simulink model "Gravity_Compensate"  (R2018b)
settings: Solver=FixedStepAuto  StartTime=0.0  StopTime=inf  FixedStep=0.001  RelTol=1e-3  EnableMultiTasking=on
values from neighbouring files (symbols this model uses):
  Dis_Coff = [0.42361 0.19319 -26.689 1.2064 -2.9972 4045.7 -3.3883 3.6846 291430]    [Robot_Parameters_Ident_With_Disturbance.mat]
  F1G = 0.2    [Main_Code.m]    (also in Main_Code_Gravity_Compensation.m)
  F2G = 0.2    [Main_Code.m]    (also in Main_Code_Gravity_Compensation.m)
  F3G = 0.005    [Main_Code.m]    (also in Main_Code_Gravity_Compensation.m)
  phi_Dynamic = [phi0;phi1;phi2;phi3;phi4;phi5;phi6;phi7]    [Parameters_Builder.m]    (also in Robot_Parameters.mat = [0.73163251 -0.0393 0 2.40643096032e-18 0.000785329049449 0.; Robot_Parameters_Ident.mat = [0.78122 -0.0393 0 2.40643096032e-18 0.000785329049449 0.000; Robot_Parameters_Ident_With_Disturbance.mat = [0.78122 -0.0393 0 2.40643096032e-18 0.000785329049449 0.000)
  phi_Kinematic = [l__0;l__1;l__3;l__5;l__2;l__7;theta;alpha;d__0;l__x35;l__z35;psi0]    [Parameters_Builder.m]    (also in Robot_Parameters.mat = [0.006 0.182 0.05 0.115 0.07 0.0342 0.733038285838 0.8726646; Robot_Parameters_Ident.mat = [0.006 0.182 0.05 0.115 0.07 0.0342 0.733038285838 0.8726646; Robot_Parameters_Ident_With_Disturbance.mat = [0.006 0.182 0.05 0.115 0.07 0.0342 0.733038285838 0.8726646)
libraries: neural x94, xpcrtudplib x3, xpcutilitieslib x2, slrtlib x1
(part 1 of 3)
settings Model: SimulationMode=external  Creator=ARAS  LastModifiedBy=ARAS
settings SolverCC: ConcurrentTasks=on  AutoInsertRateTranBlk=on
settings DataIOCC: SaveFormat=StructureWithTime
settings OptimizationCC: BlockReduction=off  OptimizeBlockIOStorage=off  BufferReuse=off  GlobalBufferReuse=off  ExpressionFolding=off  LocalBlockOutputs=off  OptimizeDataStoreBuffers=off  BusAssignmentInplaceUpdate=off
settings HardwareCC: ProdBitPerPointer=32  ProdBitPerSizeT=32  ProdBitPerPtrDiffT=32  ProdLargestAtomicFloat=None  ProdWordSize=32  ProdLongLongMode=on  ProdHWDeviceType=Generic->32-bit x86 compatible
settings RTWCC: SystemTargetFile=slrt.tlc  TemplateMakefile=slrt_default_tmf  Description=Simulink Real-Time  CodeExecutionProfiling=on  RTWCompilerOptimization=on
settings SimulinkRealTimeCC: SupportVariableSizeSignals=on  PreserveStateflowLocalDataDimensions=off  RL32LogTETModifier=off  xPCConcurrentTasks=on

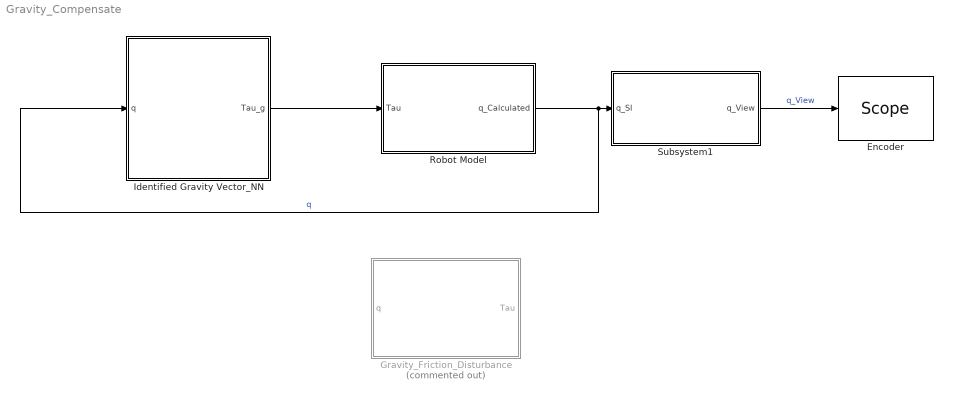
== system Gravity_Compensate ==
  Encoder : slrtlib/Displays and Logging/Scope   scopeno=2  scopetype=Target  autostart=on  viewmode=Numerical  formatstr='%15.6f'  grid=on  ylimits=[0,0]  nosamples=3  noprepostsamples=0  interleave=1  triggermode=FreeRun  triggersignal=1  trigsignalfromport=off  triggerlevel=0.0  triggerslope=Either  triggerscope=1  triggersample=0  filename=data.dat  mode=Lazy  writesize=512  autorestart=off  dynamicfilemode=off  maxwritefilesize=512*1024^2
  Gravity_Friction_Disturbance : Subsystem  Commented=on
  Identified Gravity Vector_NN : Subsystem
  Robot Model : Subsystem
  Subsystem1 : Subsystem
  wires:
  Subsystem1/1(q_View) -> Encoder/1  "q_View"
  Robot Model/1(q_Calculated) -> Identified Gravity Vector_NN/1(q), Subsystem1/1(q_SI)  "q"
  Identified Gravity Vector_NN/1(Tau_g) -> Robot Model/1(Tau)

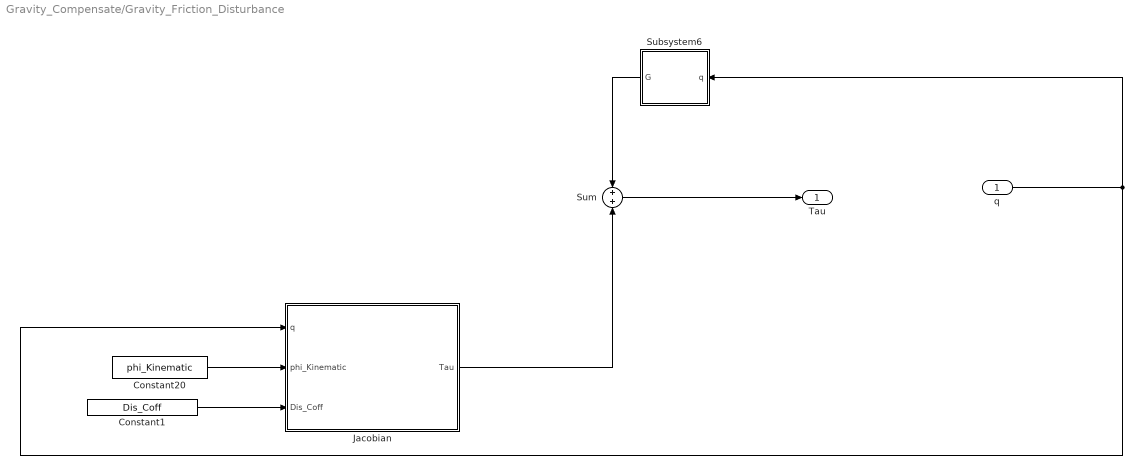
== system Gravity_Compensate/Gravity_Friction_Disturbance ==
  q : Inport
  Constant1 : Constant  Value=Dis_Coff
  Constant20 : Constant  Value=phi_Kinematic
  Jacobian : MATLAB Function  TreatAsAtomicUnit=on
  Subsystem6 : Subsystem
  Sum : Sum  Inputs=+|+
  Tau : Outport
  wires:
  q/1 -> Jacobian/1(q), Subsystem6/1(q)
  Constant1/1 -> Jacobian/3(Dis_Coff)
  Jacobian/1(Tau) -> Sum/2
  Constant20/1 -> Jacobian/2(phi_Kinematic)
  Subsystem6/1(G) -> Sum/1
  Sum/1 -> Tau/1

== system Gravity_Compensate/Identified Gravity Vector_NN ==
  q : Inport
  High_Epoch_Model : Subsystem
      mask help: Function Fitting Neural Network
      mask Display: e = 0.06;c1 = [120 150 230]/255;c2 = ([120 150 230]+0)/383;c3 = ([120 150 230]+128)/383;patch([0 1 1 0],[0 0 1 1],c1);patch([0 1 1 1-e 1-e 0+e],[0 0 1 1-e 0+e 0+e],c2);patch([0 0 1 1-e 0+e 0+e],[0 1 1 1-e 1-e 0+e],c3);plot([0 1 1 0 0],[0 0 1 1 0]);fprintf('NNET');port_label('input',1,' Input');port_label('output',1,'Output ');
  Simple_Model : Subsystem  Commented=on
      mask help: Function Fitting Neural Network
      mask Display: e = 0.06;c1 = [120 150 230]/255;c2 = ([120 150 230]+0)/383;c3 = ([120 150 230]+128)/383;patch([0 1 1 0],[0 0 1 1],c1);patch([0 1 1 1-e 1-e 0+e],[0 0 1 1-e 0+e 0+e],c2);patch([0 0 1 1-e 0+e 0+e],[0 1 1 1-e 1-e 0+e],c3);plot([0 1 1 0 0],[0 0 1 1 0]);fprintf('NNET');port_label('input',1,' Input');port_label('output',1,'Output ');
  Tau_g : Outport
  wires:
  High_Epoch_Model/1(Output) -> Tau_g/1
  q/1 -> High_Epoch_Model/1(Input)

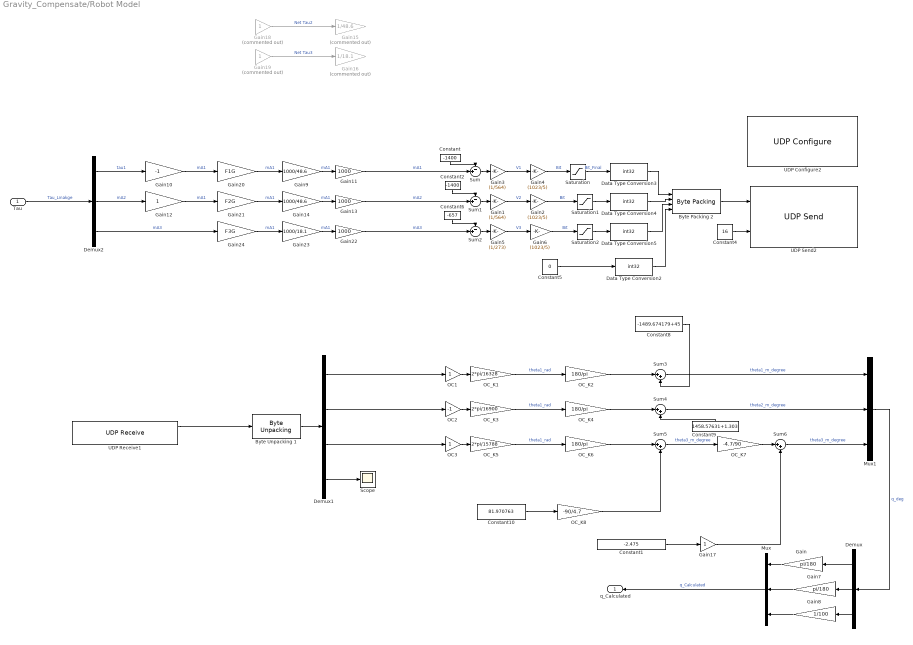
== system Gravity_Compensate/Robot Model ==
  Tau : Inport
  Byte Packing 2 : xpcutilitieslib/Byte Packing   MaskPackedDataType=uint8  MaskUnpackedDataTypes={'int32','int32','int32','int32'}  MaskAlignment=1
  Byte Unpacking 1 : xpcutilitieslib/Byte Unpacking   MaskUnpackedDataTypes={'int32'}  MaskUnpackedDataSizes={[4]}  MaskAlignment=1
      settings: SourceProductName=Simulink Real-Time  SourceProductBaseCode=XP
  Constant : Constant  Value=-1400
  Constant1 : Constant  Value=-2.475
  Constant10 : Constant  Value=81.970763
  Constant2 : Constant  Value=-1400
  Constant4 : Constant  Value=16
  Constant5 : Constant  Value=0
  Constant6 : Constant  Value=-657
  Constant8 : Constant  Value=-1489.674179+45
  Constant9 : Constant  Value=1458.57631+1.303
  Data Type Conversion{2..5} (4 alike) : DataTypeConversion  OutDataTypeStr=int32
  Demux : Demux  Outputs=3
  Demux1 : Demux
  Demux2 : Demux  Outputs=3
  Gain : Gain  Gain=pi/180
  Gain1 : Gain  Gain=(1/564)
  Gain10 : Gain  Gain=-1
  Gain11 : Gain  Gain=1000
  Gain12 : Gain
  Gain13 : Gain  Gain=1000
  Gain14 : Gain  Gain=1000/48.6
  Gain15 : Gain  Commented=on  Gain=1/48.6
  Gain16 : Gain  Commented=on  Gain=1/18.1
  Gain17 : Gain
  Gain18 : Gain  Commented=on
  Gain19 : Gain  Commented=on
  Gain2 : Gain  Gain=(1023/5)
  Gain20 : Gain  Gain=F1G
  Gain21 : Gain  Gain=F2G
  Gain22 : Gain  Gain=1000
  Gain23 : Gain  Gain=1000/18.1
  Gain24 : Gain  Gain=F3G
  Gain3 : Gain  Gain=(1/564)
  Gain4 : Gain  Gain=(1023/5)
  Gain5 : Gain  Gain=(1/273)
  Gain6 : Gain  Gain=(1023/5)
  Gain7 : Gain  Gain=pi/180
  Gain8 : Gain  Gain=1/100
  Gain9 : Gain  Gain=1000/48.6
  Mux : Mux  Inputs=3
  Mux1 : Mux  Inputs=3
  OC1 : Gain  ParamDataTypeStr=double  OutDataTypeStr=double
  OC2 : Gain  Gain=-1  ParamDataTypeStr=double  OutDataTypeStr=double
  OC3 : Gain  ParamDataTypeStr=double  OutDataTypeStr=double
  OC_K1 : Gain  Gain=2*pi/16328  ParamDataTypeStr=double  OutDataTypeStr=double
  OC_K2 : Gain  Gain=180/pi  ParamDataTypeStr=double  OutDataTypeStr=double
  OC_K3 : Gain  Gain=2*pi/16900  ParamDataTypeStr=double  OutDataTypeStr=double
  OC_K4 : Gain  Gain=180/pi  ParamDataTypeStr=double  OutDataTypeStr=double
  OC_K5 : Gain  Gain=2*pi/15788  ParamDataTypeStr=double  OutDataTypeStr=double
  OC_K6 : Gain  Gain=180/pi  ParamDataTypeStr=double  OutDataTypeStr=double
  OC_K7 : Gain  Gain=-4.7/90  ParamDataTypeStr=double  OutDataTypeStr=double
  OC_K8 : Gain  Gain=-90/4.7  ParamDataTypeStr=double  OutDataTypeStr=double
  Saturation : Saturate  UpperLimit=1023  LowerLimit=0
  Saturation1 : Saturate  UpperLimit=1023  LowerLimit=0
  Saturation2 : Saturate  UpperLimit=1023  LowerLimit=0
  Scope : Scope
  Sum : Sum  Inputs=-+|
  Sum1 : Sum  Inputs=-+|
  Sum2 : Sum  Inputs=-+|
  Sum{3..6} (4 alike) : Sum  Inputs=|++
  UDP Configure2 : xpcrtudplib/UDP Configure  Priority=-1  IpAddress=192.168.1.4  SubnetMask=255.255.255.0  Gateway=0.0.0.0  PciBus=[3]  PciSlot=[1]  PciFunction=0  ID=1  tune=0  disable=off  enableMulticast=off  MulticastIpAddress={}  MulticastMask={}
      settings: SourceProductName=Simulink Real-Time  SourceProductBaseCode=XP
  UDP Receive1 : xpcrtudplib/UDP Receive  ipAddressVal=192.168.1.4  localPort=5500  rcvWidth=16  rcvFmAny=on  fmAddress=0.0.0.0  rcvMulticast=off  multicastAddress={}  maxUDPQueue=8  sampleTime=0.001
      settings: SourceProductName=Simulink Real-Time
  UDP Send2 : xpcrtudplib/UDP Send  ipAddressVal=192.168.1.4  localPort=5500  toAddress=192.168.1.3  toPort=5500  sampleTime=0.001
      settings: SourceProductName=Simulink Real-Time  SourceProductBaseCode=XP
  q_Calculated : Outport
  wires:
  Demux1/2 -> OC2/1
  Sum/1 -> Gain3/1
  Data Type Conversion2/1 -> Byte Packing 2/4
  OC_K1/1 -> OC_K2/1  "theta1_rad"
  Byte Packing 2/1 -> UDP Send2/1
  Gain4/1 -> Saturation/1  "Bit"
  OC1/1 -> OC_K1/1
  Constant4/1 -> UDP Send2/2
  UDP Receive1/1 -> Byte Unpacking 1/1
  OC_K2/1 -> Sum3/1
  Data Type Conversion3/1 -> Byte Packing 2/1
  Data Type Conversion4/1 -> Byte Packing 2/2
  Data Type Conversion5/1 -> Byte Packing 2/3
  Demux1/3 -> OC3/1
  Constant5/1 -> Data Type Conversion2/1
  OC_K4/1 -> Sum4/1
  Constant/1 -> Sum/1
  Saturation/1 -> Data Type Conversion3/1  "Bit_Final"
  Constant10/1 -> OC_K8/1
  Gain3/1 -> Gain4/1  "V1"
  OC_K6/1 -> Sum5/1
  Saturation2/1 -> Data Type Conversion5/1
  Constant6/1 -> Sum2/1
  Gain6/1 -> Saturation2/1  "Bit"
  Gain5/1 -> Gain6/1  "V3"
  Sum2/1 -> Gain5/1
  Byte Unpacking 1/1 -> Demux1/1
  Sum1/1 -> Gain1/1
  Sum4/1 -> Mux1/2  "theta2_m_degree"
  Demux1/1 -> OC1/1
  Mux1/1 -> Demux/1  "q_deg"
  OC_K3/1 -> OC_K4/1  "theta1_rad"
  OC_K5/1 -> OC_K6/1  "theta1_rad"
  OC3/1 -> OC_K5/1
  Gain2/1 -> Saturation1/1  "Bit"
  Demux/1 -> Gain/1
  Tau/1 -> Demux2/1  "Tau_Linakge"
  Gain/1 -> Mux/1
  OC2/1 -> OC_K3/1
  Sum3/1 -> Mux1/1  "theta1_m_degree"
  Demux1/4 -> Scope/1
  Demux/2 -> Gain7/1
  Gain1/1 -> Gain2/1  "V2"
  Gain7/1 -> Mux/2
  Constant8/1 -> Sum3/2
  Constant9/1 -> Sum4/2
  Constant2/1 -> Sum1/1
  Saturation1/1 -> Data Type Conversion4/1
  Mux/1 -> q_Calculated/1  "q_Calculated"
  Gain18/1 -> Gain15/1  "Net Tau2"
  Gain19/1 -> Gain16/1  "Net Tau3"
  Demux2/1 -> Gain10/1  "tau1"
  Gain9/1 -> Gain11/1  "mA1"
  Gain10/1 -> Gain20/1  "mA1"
  Gain11/1 -> Sum/2  "mA1"
  Gain14/1 -> Gain13/1  "mA1"
  Gain12/1 -> Gain21/1  "mA1"
  Gain13/1 -> Sum1/2  "mA2"
  Demux2/2 -> Gain12/1  "mA2"
  Demux/3 -> Gain8/1
  Gain8/1 -> Mux/3
  Gain23/1 -> Gain22/1  "mA1"
  Gain22/1 -> Sum2/2  "mA3"
  Demux2/3 -> Gain24/1  "mA3"
  OC_K8/1 -> Sum5/2
  Sum5/1 -> OC_K7/1  "theta3_m_degree"
  OC_K7/1 -> Sum6/1
  Sum6/1 -> Mux1/3  "theta3_m_degree"
  Constant1/1 -> Gain17/1
  Gain17/1 -> Sum6/2
  Gain20/1 -> Gain9/1  "mA1"
  Gain21/1 -> Gain14/1  "mA1"
  Gain24/1 -> Gain23/1  "mA1"

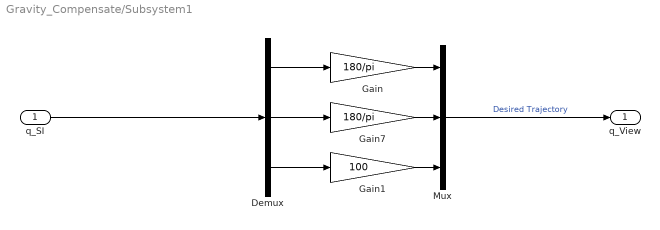
== system Gravity_Compensate/Subsystem1 ==
  q_SI : Inport
  Demux : Demux  Outputs=3
  Gain : Gain  Gain=180/pi
  Gain1 : Gain  Gain=100
  Gain7 : Gain  Gain=180/pi
  Mux : Mux  Inputs=3
  q_View : Outport
  wires:
  Gain7/1 -> Mux/2
  Demux/3 -> Gain1/1
  Demux/2 -> Gain7/1
  q_SI/1 -> Demux/1
  Gain/1 -> Mux/1
  Demux/1 -> Gain/1
  Mux/1 -> q_View/1  "Desired Trajectory"
  Gain1/1 -> Mux/3

== system Gravity_Compensate/Gravity_Friction_Disturbance/Subsystem6 ==
  q : Inport
  Constant : Constant  Value=phi_Kinematic
  Constant4 : Constant  Value=phi_Dynamic
  MATLAB Function1 : MATLAB Function  TreatAsAtomicUnit=on
  G : Outport
  wires:
  q/1 -> MATLAB Function1/1(q)
  MATLAB Function1/1(G) -> G/1
  Constant4/1 -> MATLAB Function1/3(phi_Dynamic)
  Constant/1 -> MATLAB Function1/2(phi_Kinematic)

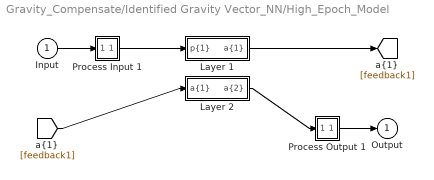
== system Gravity_Compensate/Identified Gravity Vector_NN/High_Epoch_Model ==
  Input : Inport  PortDimensions=3
      mask Display: e = 0.06;c1 = [120 230 180]/255;c2 = ([120 230 180]+0)/(256+128);c3 = ([120 230 180]+128)/(256+128);patch([0 1 1 0],[0 0 1 1],c1);patch([0 1 1 1-e 1-e 0+e],[0 0 1 1-e 0+e 0+e],c2);patch([0 0 1 1-e 0+e 0+e],[0 1 1 1-e 1-e 0+e],c3);plot([0 1 1 0 0],[0 0 1 1 0]);
  Layer 1 : Subsystem
      mask Display: e = 0.06;c1 = [120 150 230]/255;c2 = ([120 150 230]+0)/383;c3 = ([120 150 230]+128)/383;patch([0 1 1 0],[0 0 1 1],c1);patch([0 1 1 1-e 1-e 0+e],[0 0 1 1-e 0+e 0+e],c2);patch([0 0 1 1-e 0+e 0+e],[0 1 1 1-e 1-e 0+e],c3);plot([0 1 1 0 0],[0 0 1 1 0]);
  Layer 2 : Subsystem
      mask Display: e = 0.06;c1 = [120 150 230]/255;c2 = ([120 150 230]+0)/383;c3 = ([120 150 230]+128)/383;patch([0 1 1 0],[0 0 1 1],c1);patch([0 1 1 1-e 1-e 0+e],[0 0 1 1-e 0+e 0+e],c2);patch([0 0 1 1-e 0+e 0+e],[0 1 1 1-e 1-e 0+e],c3);plot([0 1 1 0 0],[0 0 1 1 0]);
  Process Input 1 : Subsystem
      mask Display: e = 0.06;c1 = [120 150 230]/255;c2 = ([120 150 230]+0)/383;c3 = ([120 150 230]+128)/383;patch([0 1 1 0],[0 0 1 1],c1);patch([0 1 1 1-e 1-e 0+e],[0 0 1 1-e 0+e 0+e],c2);patch([0 0 1 1-e 0+e 0+e],[0 1 1 1-e 1-e 0+e],c3);plot([0 1 1 0 0],[0 0 1 1 0]);
  Process Output 1 : Subsystem
      mask Display: e = 0.06;c1 = [120 150 230]/255;c2 = ([120 150 230]+0)/383;c3 = ([120 150 230]+128)/383;patch([0 1 1 0],[0 0 1 1],c1);patch([0 1 1 1-e 1-e 0+e],[0 0 1 1-e 0+e 0+e],c2);patch([0 0 1 1-e 0+e 0+e],[0 1 1 1-e 1-e 0+e],c3);plot([0 1 1 0 0],[0 0 1 1 0]);
  Output : Outport  InitialOutput=[0;0;0]
      mask Display: e = 0.06;c1 = [120 230 180]/255;c2 = ([120 230 180]+0)/(256+128);c3 = ([120 230 180]+128)/(256+128);patch([0 1 1 0],[0 0 1 1],c1);patch([0 1 1 1-e 1-e 0+e],[0 0 1 1-e 0+e 0+e],c2);patch([0 0 1 1-e 0+e 0+e],[0 1 1 1-e 1-e 0+e],c3);plot([0 1 1 0 0],[0 0 1 1 0]);
  wires:
  Input/1 -> Process Input 1/1(x)
  Process Output 1/1(y) -> Output/1
  Process Input 1/1(p) -> Layer 1/1("p{1}")
  Layer 1/1("a{1}") -> [feedback1]
  [feedback1] -> Layer 2/1("a{1} ")
  Layer 2/1("a{2}") -> Process Output 1/1(a)

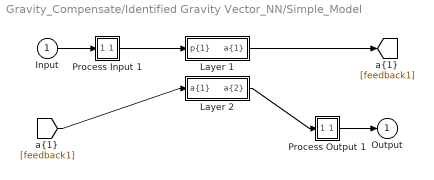
== system Gravity_Compensate/Identified Gravity Vector_NN/Simple_Model ==
  Input : Inport  PortDimensions=3
      mask Display: e = 0.06;c1 = [120 230 180]/255;c2 = ([120 230 180]+0)/(256+128);c3 = ([120 230 180]+128)/(256+128);patch([0 1 1 0],[0 0 1 1],c1);patch([0 1 1 1-e 1-e 0+e],[0 0 1 1-e 0+e 0+e],c2);patch([0 0 1 1-e 0+e 0+e],[0 1 1 1-e 1-e 0+e],c3);plot([0 1 1 0 0],[0 0 1 1 0]);
  Layer 1 : Subsystem
      mask Display: e = 0.06;c1 = [120 150 230]/255;c2 = ([120 150 230]+0)/383;c3 = ([120 150 230]+128)/383;patch([0 1 1 0],[0 0 1 1],c1);patch([0 1 1 1-e 1-e 0+e],[0 0 1 1-e 0+e 0+e],c2);patch([0 0 1 1-e 0+e 0+e],[0 1 1 1-e 1-e 0+e],c3);plot([0 1 1 0 0],[0 0 1 1 0]);
  Layer 2 : Subsystem
      mask Display: e = 0.06;c1 = [120 150 230]/255;c2 = ([120 150 230]+0)/383;c3 = ([120 150 230]+128)/383;patch([0 1 1 0],[0 0 1 1],c1);patch([0 1 1 1-e 1-e 0+e],[0 0 1 1-e 0+e 0+e],c2);patch([0 0 1 1-e 0+e 0+e],[0 1 1 1-e 1-e 0+e],c3);plot([0 1 1 0 0],[0 0 1 1 0]);
  Process Input 1 : Subsystem
      mask Display: e = 0.06;c1 = [120 150 230]/255;c2 = ([120 150 230]+0)/383;c3 = ([120 150 230]+128)/383;patch([0 1 1 0],[0 0 1 1],c1);patch([0 1 1 1-e 1-e 0+e],[0 0 1 1-e 0+e 0+e],c2);patch([0 0 1 1-e 0+e 0+e],[0 1 1 1-e 1-e 0+e],c3);plot([0 1 1 0 0],[0 0 1 1 0]);
  Process Output 1 : Subsystem
      mask Display: e = 0.06;c1 = [120 150 230]/255;c2 = ([120 150 230]+0)/383;c3 = ([120 150 230]+128)/383;patch([0 1 1 0],[0 0 1 1],c1);patch([0 1 1 1-e 1-e 0+e],[0 0 1 1-e 0+e 0+e],c2);patch([0 0 1 1-e 0+e 0+e],[0 1 1 1-e 1-e 0+e],c3);plot([0 1 1 0 0],[0 0 1 1 0]);
  Output : Outport  InitialOutput=[0;0;0]
      mask Display: e = 0.06;c1 = [120 230 180]/255;c2 = ([120 230 180]+0)/(256+128);c3 = ([120 230 180]+128)/(256+128);patch([0 1 1 0],[0 0 1 1],c1);patch([0 1 1 1-e 1-e 0+e],[0 0 1 1-e 0+e 0+e],c2);patch([0 0 1 1-e 0+e 0+e],[0 1 1 1-e 1-e 0+e],c3);plot([0 1 1 0 0],[0 0 1 1 0]);
  wires:
  Input/1 -> Process Input 1/1(x)
  Process Output 1/1(y) -> Output/1
  Process Input 1/1(p) -> Layer 1/1("p{1}")
  Layer 1/1("a{1}") -> [feedback1]
  [feedback1] -> Layer 2/1("a{1} ")
  Layer 2/1("a{2}") -> Process Output 1/1(a)

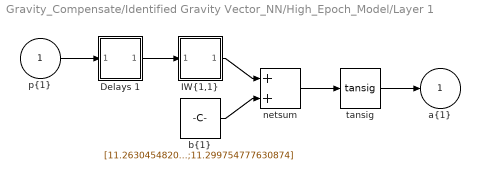
== system Gravity_Compensate/Identified Gravity Vector_NN/High_Epoch_Model/Layer 1 ==
  "p{1}" : Inport  PortDimensions=3
      mask Display: e = 0.06;c1 = [120 230 180]/255;c2 = ([120 230 180]+0)/(256+128);c3 = ([120 230 180]+128)/(256+128);patch([0 1 1 0],[0 0 1 1],c1);patch([0 1 1 1-e 1-e 0+e],[0 0 1 1-e 0+e 0+e],c2);patch([0 0 1 1-e 0+e 0+e],[0 1 1 1-e 1-e 0+e],c3);plot([0 1 1 0 0],[0 0 1 1 0]);
  Delays 1 : Subsystem
      mask Display: e = 0.06;c1 = [120 150 230]/255;c2 = ([120 150 230]+0)/383;c3 = ([120 150 230]+128)/383;patch([0 1 1 0],[0 0 1 1],c1);patch([0 1 1 1-e 1-e 0+e],[0 0 1 1-e 0+e 0+e],c2);patch([0 0 1 1-e 0+e 0+e],[0 1 1 1-e 1-e 0+e],c3);plot([0 1 1 0 0],[0 0 1 1 0]);disp('0');
  "IW{1,1}" : Subsystem
      mask Display: e = 0.06;c1 = [120 150 230]/255;c2 = ([120 150 230]+0)/383;c3 = ([120 150 230]+128)/383;patch([0 1 1 0],[0 0 1 1],c1);patch([0 1 1 1-e 1-e 0+e],[0 0 1 1-e 0+e 0+e],c2);patch([0 0 1 1-e 0+e 0+e],[0 1 1 1-e 1-e 0+e],c3);plot([0 1 1 0 0],[0 0 1 1 0]);disp('W');
  "b{1}" : Constant  Value=[11.263045482018567;6.0317742252947308;11.983996589226004;-7.6658588988543306;-5.8517886110739861;7.4451232310533406;10.917180640306658;-6.5870241683654687;8.0108681985756007;3.5513473095849979;9.6220293843375355;9.8565293533281011;3.5197166429287239;3.6957386521181124;5.6440514639510049;-3.0703225818481172;2.1993404217161325;-0.066943861917433428;-2.0448856298648423;1.6124187771848024;-0.018250185149015798;3.6417819857003435;-4.3109465870083543;-3.0890929292081832;3.9452928405896164;-5.6095743252511374;6.5578953711868264;4.3644627799494344;4.4419180604905453;7.0119603370043402;5.8581916985606002;6.7924155913571704;9.2191096669671992;-7.7729809830225198;-2.8799575409002096;-7.1021222037015077;8.151184925844742;-4.0986683409814439;9.8356397770443831;11.299754777630874]
      mask Display: e = 0.06;c1 = [120 150 230]/255;c2 = ([120 150 230]+0)/383;c3 = ([120 150 230]+128)/383;patch([0 1 1 0],[0 0 1 1],c1);patch([0 1 1 1-e 1-e 0+e],[0 0 1 1-e 0+e 0+e],c2);patch([0 0 1 1-e 0+e 0+e],[0 1 1 1-e 1-e 0+e],c3);plot([0 1 1 0 0],[0 0 1 1 0]);disp('b');
  netsum : Sum  Inputs=2  SaturateOnIntegerOverflow=on  InputSameDT=on  OutDataTypeStr=Inherit: Same as first input
      mask Display: e = 0.06;c1 = [120 150 230]/255;c2 = ([120 150 230]+0)/383;c3 = ([120 150 230]+128)/383;patch([0 1 1 0],[0 0 1 1],c1);patch([0 1 1 1-e 1-e 0+e],[0 0 1 1-e 0+e 0+e],c2);patch([0 0 1 1-e 0+e 0+e],[0 1 1 1-e 1-e 0+e],c3);plot([0 1 1 0 0],[0 0 1 1 0]);disp('+');
  tansig : neural/Transfer Functions/tansig
  "a{1}" : Outport  InitialOutput=[0;0;0;0;0;0;0;0;0;0;0;0;0;0;0;0;0;0;0;0;0;0;0;0;0;0;0;0;0;0;0;0;0;0;0;0;0;0;0;0]
      mask Display: e = 0.06;c1 = [120 230 180]/255;c2 = ([120 230 180]+0)/(256+128);c3 = ([120 230 180]+128)/(256+128);patch([0 1 1 0],[0 0 1 1],c1);patch([0 1 1 1-e 1-e 0+e],[0 0 1 1-e 0+e 0+e],c2);patch([0 0 1 1-e 0+e 0+e],[0 1 1 1-e 1-e 0+e],c3);plot([0 1 1 0 0],[0 0 1 1 0]);
  wires:
  "p{1}"/1 -> Delays 1/1("p{1}")
  Delays 1/1("pd{1,1}") -> "IW{1,1}"/1("pd{1,1}")
  "IW{1,1}"/1("iz{1,1}") -> netsum/1
  "b{1}"/1 -> netsum/2
  netsum/1 -> tansig/1
  tansig/1 -> "a{1}"/1

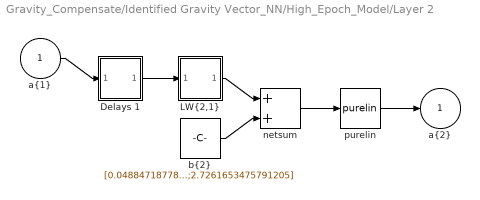
== system Gravity_Compensate/Identified Gravity Vector_NN/High_Epoch_Model/Layer 2 ==
  "a{1} " : Inport  PortDimensions=40
      mask Display: e = 0.06;c1 = [120 230 180]/255;c2 = ([120 230 180]+0)/(256+128);c3 = ([120 230 180]+128)/(256+128);patch([0 1 1 0],[0 0 1 1],c1);patch([0 1 1 1-e 1-e 0+e],[0 0 1 1-e 0+e 0+e],c2);patch([0 0 1 1-e 0+e 0+e],[0 1 1 1-e 1-e 0+e],c3);plot([0 1 1 0 0],[0 0 1 1 0]);
  Delays 1 : Subsystem
      mask Display: e = 0.06;c1 = [120 150 230]/255;c2 = ([120 150 230]+0)/383;c3 = ([120 150 230]+128)/383;patch([0 1 1 0],[0 0 1 1],c1);patch([0 1 1 1-e 1-e 0+e],[0 0 1 1-e 0+e 0+e],c2);patch([0 0 1 1-e 0+e 0+e],[0 1 1 1-e 1-e 0+e],c3);plot([0 1 1 0 0],[0 0 1 1 0]);disp('0');
  "LW{2,1}" : Subsystem
      mask Display: e = 0.06;c1 = [120 150 230]/255;c2 = ([120 150 230]+0)/383;c3 = ([120 150 230]+128)/383;patch([0 1 1 0],[0 0 1 1],c1);patch([0 1 1 1-e 1-e 0+e],[0 0 1 1-e 0+e 0+e],c2);patch([0 0 1 1-e 0+e 0+e],[0 1 1 1-e 1-e 0+e],c3);plot([0 1 1 0 0],[0 0 1 1 0]);disp('W');
  "b{2}" : Constant  Value=[0.048847187789358953;-0.86208257404274102;2.7261653475791205]
      mask Display: e = 0.06;c1 = [120 150 230]/255;c2 = ([120 150 230]+0)/383;c3 = ([120 150 230]+128)/383;patch([0 1 1 0],[0 0 1 1],c1);patch([0 1 1 1-e 1-e 0+e],[0 0 1 1-e 0+e 0+e],c2);patch([0 0 1 1-e 0+e 0+e],[0 1 1 1-e 1-e 0+e],c3);plot([0 1 1 0 0],[0 0 1 1 0]);disp('b');
  netsum : Sum  Inputs=2  SaturateOnIntegerOverflow=on  InputSameDT=on  OutDataTypeStr=Inherit: Same as first input
      mask Display: e = 0.06;c1 = [120 150 230]/255;c2 = ([120 150 230]+0)/383;c3 = ([120 150 230]+128)/383;patch([0 1 1 0],[0 0 1 1],c1);patch([0 1 1 1-e 1-e 0+e],[0 0 1 1-e 0+e 0+e],c2);patch([0 0 1 1-e 0+e 0+e],[0 1 1 1-e 1-e 0+e],c3);plot([0 1 1 0 0],[0 0 1 1 0]);disp('+');
  purelin : neural/Transfer Functions/purelin
  "a{2}" : Outport  InitialOutput=[0;0;0]
      mask Display: e = 0.06;c1 = [120 230 180]/255;c2 = ([120 230 180]+0)/(256+128);c3 = ([120 230 180]+128)/(256+128);patch([0 1 1 0],[0 0 1 1],c1);patch([0 1 1 1-e 1-e 0+e],[0 0 1 1-e 0+e 0+e],c2);patch([0 0 1 1-e 0+e 0+e],[0 1 1 1-e 1-e 0+e],c3);plot([0 1 1 0 0],[0 0 1 1 0]);
  wires:
  "a{1} "/1 -> Delays 1/1("p{2}")
  Delays 1/1("pd{2,1}") -> "LW{2,1}"/1("ad{2,1}")
  "LW{2,1}"/1("lz{2,1}") -> netsum/1
  "b{2}"/1 -> netsum/2
  netsum/1 -> purelin/1
  purelin/1 -> "a{2}"/1

== system Gravity_Compensate/Identified Gravity Vector_NN/High_Epoch_Model/Process Input 1 ==
  x : Inport  PortDimensions=3
      mask Display: e = 0.06;c1 = [120 230 180]/255;c2 = ([120 230 180]+0)/(256+128);c3 = ([120 230 180]+128)/(256+128);patch([0 1 1 0],[0 0 1 1],c1);patch([0 1 1 1-e 1-e 0+e],[0 0 1 1-e 0+e 0+e],c2);patch([0 0 1 1-e 0+e 0+e],[0 1 1 1-e 1-e 0+e],c3);plot([0 1 1 0 0],[0 0 1 1 0]);
  mapminmax : neural/Processing Functions/mapminmax  xmin=[-0.74119943464489935;-0.38317773452897713;-0.021732938110557955]  xmax=[0.73970195514479398;1.1328739374495371;0.013612498803619413]  ymin=-1  ymax=1
  p : Outport  PortDimensions=3
      mask Display: e = 0.06;c1 = [120 230 180]/255;c2 = ([120 230 180]+0)/(256+128);c3 = ([120 230 180]+128)/(256+128);patch([0 1 1 0],[0 0 1 1],c1);patch([0 1 1 1-e 1-e 0+e],[0 0 1 1-e 0+e 0+e],c2);patch([0 0 1 1-e 0+e 0+e],[0 1 1 1-e 1-e 0+e],c3);plot([0 1 1 0 0],[0 0 1 1 0]);
  wires:
  x/1 -> mapminmax/1
  mapminmax/1 -> p/1

== system Gravity_Compensate/Identified Gravity Vector_NN/High_Epoch_Model/Process Output 1 ==
  a : Inport  PortDimensions=3
      mask Display: e = 0.06;c1 = [120 230 180]/255;c2 = ([120 230 180]+0)/(256+128);c3 = ([120 230 180]+128)/(256+128);patch([0 1 1 0],[0 0 1 1],c1);patch([0 1 1 1-e 1-e 0+e],[0 0 1 1-e 0+e 0+e],c2);patch([0 0 1 1-e 0+e 0+e],[0 1 1 1-e 1-e 0+e],c3);plot([0 1 1 0 0],[0 0 1 1 0]);
  mapminmax_reverse : neural/Processing Functions/mapminmax_reverse  xmin=[-0.033440063296072985;-0.32275006138566892;-1.0286523309339672]  xmax=[0.063380196443186279;0.12759754131993545;2.2684770577140809]  ymin=-1  ymax=1
  y : Outport  PortDimensions=3
      mask Display: e = 0.06;c1 = [120 230 180]/255;c2 = ([120 230 180]+0)/(256+128);c3 = ([120 230 180]+128)/(256+128);patch([0 1 1 0],[0 0 1 1],c1);patch([0 1 1 1-e 1-e 0+e],[0 0 1 1-e 0+e 0+e],c2);patch([0 0 1 1-e 0+e 0+e],[0 1 1 1-e 1-e 0+e],c3);plot([0 1 1 0 0],[0 0 1 1 0]);
  wires:
  a/1 -> mapminmax_reverse/1
  mapminmax_reverse/1 -> y/1

== system Gravity_Compensate/Identified Gravity Vector_NN/Simple_Model/Layer 1 ==
  "p{1}" : Inport  PortDimensions=3
      mask Display: e = 0.06;c1 = [120 230 180]/255;c2 = ([120 230 180]+0)/(256+128);c3 = ([120 230 180]+128)/(256+128);patch([0 1 1 0],[0 0 1 1],c1);patch([0 1 1 1-e 1-e 0+e],[0 0 1 1-e 0+e 0+e],c2);patch([0 0 1 1-e 0+e 0+e],[0 1 1 1-e 1-e 0+e],c3);plot([0 1 1 0 0],[0 0 1 1 0]);
  Delays 1 : Subsystem
      mask Display: e = 0.06;c1 = [120 150 230]/255;c2 = ([120 150 230]+0)/383;c3 = ([120 150 230]+128)/383;patch([0 1 1 0],[0 0 1 1],c1);patch([0 1 1 1-e 1-e 0+e],[0 0 1 1-e 0+e 0+e],c2);patch([0 0 1 1-e 0+e 0+e],[0 1 1 1-e 1-e 0+e],c3);plot([0 1 1 0 0],[0 0 1 1 0]);disp('0');
  "IW{1,1}" : Subsystem
      mask Display: e = 0.06;c1 = [120 150 230]/255;c2 = ([120 150 230]+0)/383;c3 = ([120 150 230]+128)/383;patch([0 1 1 0],[0 0 1 1],c1);patch([0 1 1 1-e 1-e 0+e],[0 0 1 1-e 0+e 0+e],c2);patch([0 0 1 1-e 0+e 0+e],[0 1 1 1-e 1-e 0+e],c3);plot([0 1 1 0 0],[0 0 1 1 0]);disp('W');
  "b{1}" : Constant  Value=[-5.1671024702432309;-4.5492478496736481;6.3513007169439613;-4.3242169443066025;-4.9099577859238943;2.9884422969247351;2.8596984211429541;-3.7229427812616276;-4.0428021820626672;-3.8857383513373862;2.9200064524284417;-2.6645569397562268;-1.7204116061242201;2.014594232626655;-0.35961089589387885;-0.2621781845842307;1.3946786816292078;-0.97621350752330682;0.228894699065709;0.033846042744305874;0.19550889877932565;-0.22048224192437449;0.84308806787731638;1.0060244602223873;1.2805122000397808;1.8992799952460735;1.6540344435035461;-2.3422673285028055;2.3237871742652998;-3.0449307864880586;4.107231896059667;-2.962271952856887;-3.1024467734324115;-3.5747733282385905;-3.7885684814460707;3.7783425802523833;4.4237939827471164;-5.7418357373864728;5.4040784348450339;-5.686679084330482]
      mask Display: e = 0.06;c1 = [120 150 230]/255;c2 = ([120 150 230]+0)/383;c3 = ([120 150 230]+128)/383;patch([0 1 1 0],[0 0 1 1],c1);patch([0 1 1 1-e 1-e 0+e],[0 0 1 1-e 0+e 0+e],c2);patch([0 0 1 1-e 0+e 0+e],[0 1 1 1-e 1-e 0+e],c3);plot([0 1 1 0 0],[0 0 1 1 0]);disp('b');
  netsum : Sum  Inputs=2  SaturateOnIntegerOverflow=on  InputSameDT=on  OutDataTypeStr=Inherit: Same as first input
      mask Display: e = 0.06;c1 = [120 150 230]/255;c2 = ([120 150 230]+0)/383;c3 = ([120 150 230]+128)/383;patch([0 1 1 0],[0 0 1 1],c1);patch([0 1 1 1-e 1-e 0+e],[0 0 1 1-e 0+e 0+e],c2);patch([0 0 1 1-e 0+e 0+e],[0 1 1 1-e 1-e 0+e],c3);plot([0 1 1 0 0],[0 0 1 1 0]);disp('+');
  tansig : neural/Transfer Functions/tansig
  "a{1}" : Outport  InitialOutput=[0;0;0;0;0;0;0;0;0;0;0;0;0;0;0;0;0;0;0;0;0;0;0;0;0;0;0;0;0;0;0;0;0;0;0;0;0;0;0;0]
      mask Display: e = 0.06;c1 = [120 230 180]/255;c2 = ([120 230 180]+0)/(256+128);c3 = ([120 230 180]+128)/(256+128);patch([0 1 1 0],[0 0 1 1],c1);patch([0 1 1 1-e 1-e 0+e],[0 0 1 1-e 0+e 0+e],c2);patch([0 0 1 1-e 0+e 0+e],[0 1 1 1-e 1-e 0+e],c3);plot([0 1 1 0 0],[0 0 1 1 0]);
  wires:
  "p{1}"/1 -> Delays 1/1("p{1}")
  Delays 1/1("pd{1,1}") -> "IW{1,1}"/1("pd{1,1}")
  "IW{1,1}"/1("iz{1,1}") -> netsum/1
  "b{1}"/1 -> netsum/2
  netsum/1 -> tansig/1
  tansig/1 -> "a{1}"/1

== system Gravity_Compensate/Identified Gravity Vector_NN/Simple_Model/Layer 2 ==
  "a{1} " : Inport  PortDimensions=40
      mask Display: e = 0.06;c1 = [120 230 180]/255;c2 = ([120 230 180]+0)/(256+128);c3 = ([120 230 180]+128)/(256+128);patch([0 1 1 0],[0 0 1 1],c1);patch([0 1 1 1-e 1-e 0+e],[0 0 1 1-e 0+e 0+e],c2);patch([0 0 1 1-e 0+e 0+e],[0 1 1 1-e 1-e 0+e],c3);plot([0 1 1 0 0],[0 0 1 1 0]);
  Delays 1 : Subsystem
      mask Display: e = 0.06;c1 = [120 150 230]/255;c2 = ([120 150 230]+0)/383;c3 = ([120 150 230]+128)/383;patch([0 1 1 0],[0 0 1 1],c1);patch([0 1 1 1-e 1-e 0+e],[0 0 1 1-e 0+e 0+e],c2);patch([0 0 1 1-e 0+e 0+e],[0 1 1 1-e 1-e 0+e],c3);plot([0 1 1 0 0],[0 0 1 1 0]);disp('0');
  "LW{2,1}" : Subsystem
      mask Display: e = 0.06;c1 = [120 150 230]/255;c2 = ([120 150 230]+0)/383;c3 = ([120 150 230]+128)/383;patch([0 1 1 0],[0 0 1 1],c1);patch([0 1 1 1-e 1-e 0+e],[0 0 1 1-e 0+e 0+e],c2);patch([0 0 1 1-e 0+e 0+e],[0 1 1 1-e 1-e 0+e],c3);plot([0 1 1 0 0],[0 0 1 1 0]);disp('W');
  "b{2}" : Constant  Value=[-0.75793513529392142;-0.23015719052432385;-0.35793819882989186]
      mask Display: e = 0.06;c1 = [120 150 230]/255;c2 = ([120 150 230]+0)/383;c3 = ([120 150 230]+128)/383;patch([0 1 1 0],[0 0 1 1],c1);patch([0 1 1 1-e 1-e 0+e],[0 0 1 1-e 0+e 0+e],c2);patch([0 0 1 1-e 0+e 0+e],[0 1 1 1-e 1-e 0+e],c3);plot([0 1 1 0 0],[0 0 1 1 0]);disp('b');
  netsum : Sum  Inputs=2  SaturateOnIntegerOverflow=on  InputSameDT=on  OutDataTypeStr=Inherit: Same as first input
      mask Display: e = 0.06;c1 = [120 150 230]/255;c2 = ([120 150 230]+0)/383;c3 = ([120 150 230]+128)/383;patch([0 1 1 0],[0 0 1 1],c1);patch([0 1 1 1-e 1-e 0+e],[0 0 1 1-e 0+e 0+e],c2);patch([0 0 1 1-e 0+e 0+e],[0 1 1 1-e 1-e 0+e],c3);plot([0 1 1 0 0],[0 0 1 1 0]);disp('+');
  purelin : neural/Transfer Functions/purelin
  "a{2}" : Outport  InitialOutput=[0;0;0]
      mask Display: e = 0.06;c1 = [120 230 180]/255;c2 = ([120 230 180]+0)/(256+128);c3 = ([120 230 180]+128)/(256+128);patch([0 1 1 0],[0 0 1 1],c1);patch([0 1 1 1-e 1-e 0+e],[0 0 1 1-e 0+e 0+e],c2);patch([0 0 1 1-e 0+e 0+e],[0 1 1 1-e 1-e 0+e],c3);plot([0 1 1 0 0],[0 0 1 1 0]);
  wires:
  "a{1} "/1 -> Delays 1/1("p{2}")
  Delays 1/1("pd{2,1}") -> "LW{2,1}"/1("ad{2,1}")
  "LW{2,1}"/1("lz{2,1}") -> netsum/1
  "b{2}"/1 -> netsum/2
  netsum/1 -> purelin/1
  purelin/1 -> "a{2}"/1

== system Gravity_Compensate/Identified Gravity Vector_NN/Simple_Model/Process Input 1 ==
  x : Inport  PortDimensions=3
      mask Display: e = 0.06;c1 = [120 230 180]/255;c2 = ([120 230 180]+0)/(256+128);c3 = ([120 230 180]+128)/(256+128);patch([0 1 1 0],[0 0 1 1],c1);patch([0 1 1 1-e 1-e 0+e],[0 0 1 1-e 0+e 0+e],c2);patch([0 0 1 1-e 0+e 0+e],[0 1 1 1-e 1-e 0+e],c3);plot([0 1 1 0 0],[0 0 1 1 0]);
  mapminmax : neural/Processing Functions/mapminmax  xmin=[-0.74119943464489935;-0.38317773452897713;-0.021732938110557955]  xmax=[0.73970195514479398;1.1328739374495371;0.013612498803619413]  ymin=-1  ymax=1
  p : Outport  PortDimensions=3
      mask Display: e = 0.06;c1 = [120 230 180]/255;c2 = ([120 230 180]+0)/(256+128);c3 = ([120 230 180]+128)/(256+128);patch([0 1 1 0],[0 0 1 1],c1);patch([0 1 1 1-e 1-e 0+e],[0 0 1 1-e 0+e 0+e],c2);patch([0 0 1 1-e 0+e 0+e],[0 1 1 1-e 1-e 0+e],c3);plot([0 1 1 0 0],[0 0 1 1 0]);
  wires:
  x/1 -> mapminmax/1
  mapminmax/1 -> p/1

== system Gravity_Compensate/Identified Gravity Vector_NN/Simple_Model/Process Output 1 ==
  a : Inport  PortDimensions=3
      mask Display: e = 0.06;c1 = [120 230 180]/255;c2 = ([120 230 180]+0)/(256+128);c3 = ([120 230 180]+128)/(256+128);patch([0 1 1 0],[0 0 1 1],c1);patch([0 1 1 1-e 1-e 0+e],[0 0 1 1-e 0+e 0+e],c2);patch([0 0 1 1-e 0+e 0+e],[0 1 1 1-e 1-e 0+e],c3);plot([0 1 1 0 0],[0 0 1 1 0]);
  mapminmax_reverse : neural/Processing Functions/mapminmax_reverse  xmin=[-0.033440063296072985;-0.32275006138566892;-1.0286523309339672]  xmax=[0.063380196443186279;0.12759754131993545;2.2684770577140809]  ymin=-1  ymax=1
  y : Outport  PortDimensions=3
      mask Display: e = 0.06;c1 = [120 230 180]/255;c2 = ([120 230 180]+0)/(256+128);c3 = ([120 230 180]+128)/(256+128);patch([0 1 1 0],[0 0 1 1],c1);patch([0 1 1 1-e 1-e 0+e],[0 0 1 1-e 0+e 0+e],c2);patch([0 0 1 1-e 0+e 0+e],[0 1 1 1-e 1-e 0+e],c3);plot([0 1 1 0 0],[0 0 1 1 0]);
  wires:
  a/1 -> mapminmax_reverse/1
  mapminmax_reverse/1 -> y/1

== system Gravity_Compensate/Identified Gravity Vector_NN/High_Epoch_Model/Layer 1/Delays 1 ==
  "p{1}" : Inport  PortDimensions=3
      mask Display: e = 0.06;c1 = [120 230 180]/255;c2 = ([120 230 180]+0)/(256+128);c3 = ([120 230 180]+128)/(256+128);patch([0 1 1 0],[0 0 1 1],c1);patch([0 1 1 1-e 1-e 0+e],[0 0 1 1-e 0+e 0+e],c2);patch([0 0 1 1-e 0+e 0+e],[0 1 1 1-e 1-e 0+e],c3);plot([0 1 1 0 0],[0 0 1 1 0]);
  mux : Mux  Inputs=1
      mask Display: e = 0.06;c1 = [120 150 230]/255;c2 = ([120 150 230]+0)/383;c3 = ([120 150 230]+128)/383;patch([0 1 1 0],[0 0 1 1],c1);patch([0 1 1 1-e 1-e 0+e],[0 0 1 1-e 0+e 0+e],c2);patch([0 0 1 1-e 0+e 0+e],[0 1 1 1-e 1-e 0+e],c3);plot([0 1 1 0 0],[0 0 1 1 0]);disp('Mux')
  "pd{1,1}" : Outport
      mask Display: e = 0.06;c1 = [120 230 180]/255;c2 = ([120 230 180]+0)/(256+128);c3 = ([120 230 180]+128)/(256+128);patch([0 1 1 0],[0 0 1 1],c1);patch([0 1 1 1-e 1-e 0+e],[0 0 1 1-e 0+e 0+e],c2);patch([0 0 1 1-e 0+e 0+e],[0 1 1 1-e 1-e 0+e],c3);plot([0 1 1 0 0],[0 0 1 1 0]);
  wires:
  "p{1}"/1 -> mux/1
  mux/1 -> "pd{1,1}"/1
